simulink model "SupervisorB2"  (R2024b)
settings: Solver=FixedStepDiscrete  StartTime=0.0  StopTime=10.0  FixedStep=0.02  RelTol=1e-3
settings Model: DataDictionary=B2Sup.sldd  PacingRate=0.100000  Creator=miche  LastModifiedBy=Sterm
settings OptimizationCC: DefaultParameterBehavior=Inlined  EnhancedBackFolding=on  PassReuseOutputArgsAs=Individual arguments  ZeroExternalMemoryAtStartup=off  ZeroInternalMemoryAtStartup=off  OptimizeBlockOrder=speed  DifferentSizesBufferReuse=on  OptimizationCustomize=off  EfficientTunableParamExpr=on
settings DebuggingCC: ParameterTunabilityLossMsg=error
settings SFSimCC: MATLABDynamicMemAlloc=off
settings SFSimCC: SimUserIncludeDirs=|
  | C:\Users\Sterm\Desktop\STM32\workspace\Codice_Rover
  | C:\Users\Sterm\Desktop\STM32\workspace\Codice_Rover\Progetto_Board2\Core\Inc
settings RTWCC: Description=Embedded Coder  SystemTargetFile=ert.tlc  GenCodeOnly=on  TemplateMakefile=ert_default_tmf
settings CodeAppCC: ForceParamTrailComments=on  IgnoreCustomStorageClasses=off  OperatorAnnotations=on  SimulinkDataObjDesc=on  SFDataObjDesc=on  InsertBlockDesc=on
settings ERTTargetCC: TargetLangStandard=C99 (ISO)  GenerateSampleERTMain=on  ERTCustomFileTemplate=example_file_process.tlc

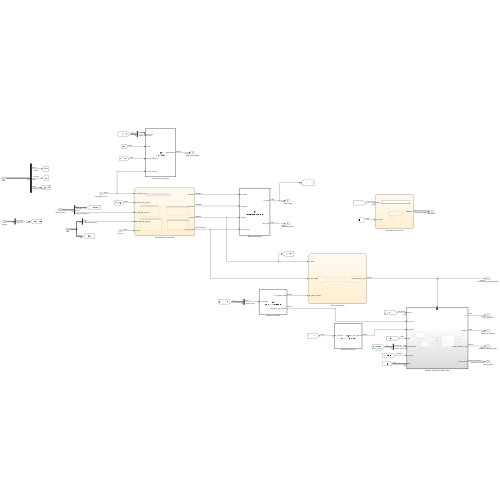
[thumbnail: Simulink's stored preview of the top-level diagram]
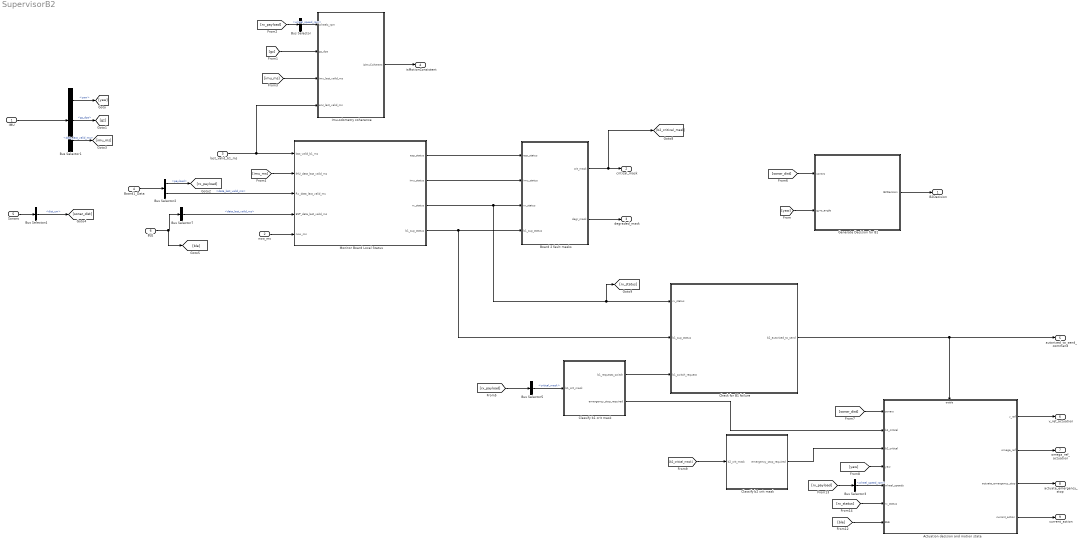
== system SupervisorB2 ==
  IMU : Inport  OutDataTypeStr=Bus: IMUSnapshot_t
  now_ms : Inport  Port=2  OutDataTypeStr=uint32
  last_valid_b1_ms : Inport  Port=3  OutDataTypeStr=uint32
  Board1_Data : Inport  Port=4  OutDataTypeStr=Bus: RxSnapshot_t
  Sonars : Inport  Port=5  OutDataTypeStr=Bus: SonarSnapshot_t
  BLE : Inport  Port=6  OutDataTypeStr=Bus: BleControllerSnapshot_t
  Actuation decision and motion state : Subsystem  TreatAsAtomicUnit=on
  Board 2 fault masks : MATLAB Function  TreatAsAtomicUnit=on
  Bus Selector : BusSelector  OutputSignals=wheel_speed_rpm
  Bus Selector1 : BusSelector  OutputSignals=yaw,gz_dps,data_last_valid_ms
  Bus Selector2 : BusSelector  OutputSignals=payload,data_last_valid_ms
  Bus Selector3 : BusSelector  OutputSignals=wheel_speed_rpm
  Bus Selector4 : BusSelector  OutputSignals=dist_cm
  Bus Selector5 : BusSelector  OutputSignals=critical_mask
  Bus Selector7 : BusSelector  OutputSignals=data_last_valid_ms
  Check for B1 failure : Stateflow chart  TreatAsAtomicUnit=on
      settings: RTWFcnNameOpts=Use subsystem name  RTWFileNameOpts=Use subsystem name  PortSchema="{\"entries\":[{\"content\":{\"sides\":[{\"content\":{\"connectorIds\":[\"In2\",\"In3\",\"In1\"]},\"type\":\"ConnectorPlacement.EquallySpacedRectSide\",\"uuid\":\"67b49e78-6b94-400e-9fcc-b30b67a80691\"},{\"content\":{\"connectorIds\":[\"Out1\"],\"side\":\"RIGHT\"},\"type\":\"ConnectorPlacement.EquallySpacedRectSide\",\"uuid\":\"f9efb856-d575-4b84-9867-a72704ddd64e\"},{\"content\":{\"side\":\"TOP\"},\"type\":\"ConnectorPlacement.EquallySpacedRectSide\",\"uuid\":\"fb0179cd-4de4-48aa-8472-d7b382cb3b22\"}]},\"type\":\"ConnectorPlacement.EquallySpacedConnector\",\"uuid\":\"a3077d23-e6fe-47c9-9a8f-de3eab952316\"}],\"packageUris\":[\"http://schema.mathworks.com/mf0/Connector/R2020b\"],\"version\":\"1.0\"}"
  Classify b1 crit mask : MATLAB Function  TreatAsAtomicUnit=on
  Classify b2 crit mask : MATLAB Function  TreatAsAtomicUnit=on
  Generate Decision for B1 : Stateflow chart  TreatAsAtomicUnit=on
      settings: RTWFcnNameOpts=Use subsystem name  RTWFileNameOpts=Use subsystem name
  Imu-odometry coherence : MATLAB Function  TreatAsAtomicUnit=on
  Monitor Board Local Status : Stateflow chart  TreatAsAtomicUnit=on
      settings: PortSchema="{\"entries\":[{\"content\":{\"sides\":[{\"content\":{\"connectorIds\":[\"In3\",\"In1\",\"In4\",\"In5\",\"In2\"]},\"type\":\"ConnectorPlacement.EquallySpacedRectSide\",\"uuid\":\"47aaac17-a3c1-4cfa-9019-2fc909ce8afb\"},{\"content\":{\"connectorIds\":[\"Out4\",\"Out2\",\"Out3\",\"Out1\"],\"side\":\"RIGHT\"},\"type\":\"ConnectorPlacement.EquallySpacedRectSide\",\"uuid\":\"50480d75-ffb6-4b14-98f4-247cb8499fa0\"},{\"content\":{\"side\":\"TOP\"},\"type\":\"ConnectorPlacement.EquallySpacedRectSide\",\"uuid\":\"1cb4b11b-b488-43f8-b4d2-41a29965dbbd\"}]},\"type\":\"ConnectorPlacement.EquallySpacedConnector\",\"uuid\":\"f85d8103-6e2e-468d-83b6-a974a06ba402\"}],\"packageUris\":[\"http://schema.mathworks.com/mf0/Connector/R2020b\"],\"version\":\"1.0\"}"
  B2Decision : Outport  OutDataTypeStr=Enum: SupervisorCommand_t  PortDimensions=1
  critical_mask : Outport  Port=2  OutDataTypeStr=uint32
  degraded_mask : Outport  Port=3  OutDataTypeStr=uint32
  isMotionConsistent : Outport  Port=4  OutDataTypeStr=boolean
  autorized_to_send_command : Outport  Port=5  OutDataTypeStr=boolean  PortDimensions=1
  v_ref_actuation : Outport  Port=6  OutDataTypeStr=single  PortDimensions=1
  omega_ref_actuation : Outport  Port=7  OutDataTypeStr=single  PortDimensions=1
  actuate_emergency_stop : Outport  Port=8  OutDataTypeStr=boolean
  current_action : Outport  Port=9  OutDataTypeStr=Enum: SupervisorCommand_t
  wires:
  Bus Selector1/1 -> [yaw]  "<yaw>"
  Board1_Data/1 -> Bus Selector2/1
  Bus Selector2/2 -> Monitor Board Local Status/4(Rx_data_last_valid_ms)  "<data_last_valid_ms>"
  Generate Decision for B1/1(B2Decision) -> B2Decision/1
  Monitor Board Local Status/2(imu_status) -> Board 2 fault masks/2(imu_status)
  last_valid_b1_ms/1 -> Monitor Board Local Status/3(last_valid_b1_ms), Imu-odometry coherence/4(enc_last_valid_ms)
  now_ms/1 -> Monitor Board Local Status/2(now_ms)
  Board 2 fault masks/1(crit_mask) -> [b2_critical_mask], critical_mask/1
  IMU/1 -> Bus Selector1/1
  Imu-odometry coherence/1(isImuCoherent) -> isMotionConsistent/1
  [sonar_dist] -> Generate Decision for B1/1(sonars)
  Monitor Board Local Status/1(b1_sup_status) -> Check for B1 failure/3(b1_sup_status), Board 2 fault masks/4(b1_sup_status)
  [yaw] -> Generate Decision for B1/2(gyro_angle)
  Board 2 fault masks/2(degr_mask) -> degraded_mask/1
  Bus Selector1/2 -> [gz]  "<gz_dps>"
  Monitor Board Local Status/4(esp_status) -> Board 2 fault masks/1(esp_status)
  Monitor Board Local Status/3(rx_status) -> Check for B1 failure/2(rx_status), [rx_status], Board 2 fault masks/3(rx_status)
  [gz] -> Imu-odometry coherence/2(gz_dps)
  [rx_payload] -> Bus Selector/1
  Bus Selector1/3 -> [imu_ms]  "<data_last_valid_ms>"
  [imu_ms] -> Imu-odometry coherence/3(imu_last_valid_ms)
  [imu_ms] -> Monitor Board Local Status/1(IMU_data_last_valid_ms)
  Bus Selector2/1 -> [rx_payload]  "<payload>"
  Bus Selector/1 -> Imu-odometry coherence/1(wheels_rpm)  "<wheel_speed_rpm>"
  [rx_payload] -> Bus Selector5/1
  Bus Selector5/1 -> Classify b1 crit mask/1(b1_crit_mask)  "<critical_mask>"
  Classify b1 crit mask/1(b1_requests_switch) -> Check for B1 failure/1(b1_switch_request)
  Classify b1 crit mask/2(emergency_stop_required) -> Actuation decision and motion state/2(b1_critical)
  Check for B1 failure/1(b2_autorized_to_send) -> Actuation decision and motion state/Enable, autorized_to_send_command/1
  Sonars/1 -> Bus Selector4/1
  Bus Selector4/1 -> [sonar_dist]  "<dist_cm>"
  [sonar_dist] -> Actuation decision and motion state/1(sonars)
  [yaw] -> Actuation decision and motion state/4(yaw)
  BLE/1 -> [ble], Bus Selector7/1
  Bus Selector7/1 -> Monitor Board Local Status/5(ESP_data_last_valid_ms)  "<data_last_valid_ms>"
  [ble] -> Actuation decision and motion state/7(BLE)
  [b2_critical_mask] -> Classify b2 crit mask/1(b2_crit_mask)
  Classify b2 crit mask/1(emergency_stop_required) -> Actuation decision and motion state/3(b2_critical)
  Actuation decision and motion state/1(v_ref) -> v_ref_actuation/1
  Actuation decision and motion state/2(omega_ref) -> omega_ref_actuation/1
  Bus Selector3/1 -> Actuation decision and motion state/5(wheel_speeds)  "<wheel_speed_rpm>"
  [rx_payload] -> Bus Selector3/1
  [rx_status] -> Actuation decision and motion state/6(rx_status)
  Actuation decision and motion state/3(actuate_emergency_stop) -> actuate_emergency_stop/1
  Actuation decision and motion state/4(current_action) -> current_action/1

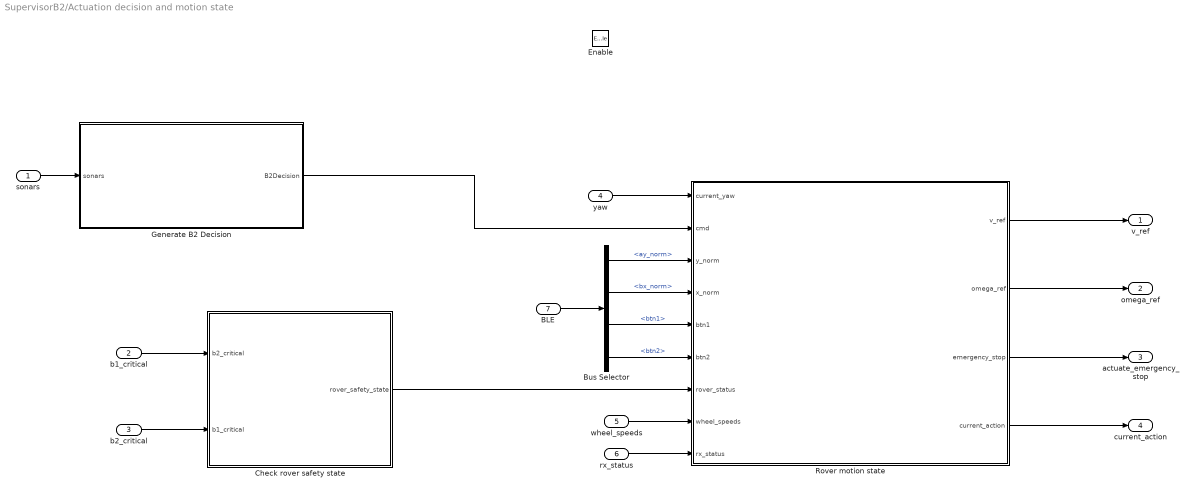
== system SupervisorB2/Actuation decision and motion state ==
  sonars : Inport
  b1_critical : Inport  Port=2
  b2_critical : Inport  Port=3
  yaw : Inport  Port=4
  wheel_speeds : Inport  Port=5
  rx_status : Inport  Port=6
  BLE : Inport  Port=7
  Enable : EnablePort
  Bus Selector : BusSelector  OutputSignals=ay_norm,bx_norm,btn1,btn2
  Check rover safety state : Stateflow chart  TreatAsAtomicUnit=on
      settings: PortSchema="{\"entries\":[{\"content\":{\"sides\":[{\"content\":{\"connectorIds\":[\"In2\",\"In1\"]},\"type\":\"ConnectorPlacement.EquallySpacedRectSide\",\"uuid\":\"9dc33dbe-e010-4406-a301-8909eb6c65d2\"},{\"content\":{\"connectorIds\":[\"Out1\"],\"side\":\"RIGHT\"},\"type\":\"ConnectorPlacement.EquallySpacedRectSide\",\"uuid\":\"084d7bfb-fdfa-425b-9b48-9ea13f8992e6\"},{\"content\":{\"side\":\"TOP\"},\"type\":\"ConnectorPlacement.EquallySpacedRectSide\",\"uuid\":\"e02a7452-bac4-4562-b32b-e5d8b54b8354\"}]},\"type\":\"ConnectorPlacement.EquallySpacedConnector\",\"uuid\":\"22e5b97d-2191-437a-a89c-d8bb13bb1f1c\"}],\"packageUris\":[\"http://schema.mathworks.com/mf0/Connector/R2020b\"],\"version\":\"1.0\"}"
  Generate B2 Decision : Stateflow chart  TreatAsAtomicUnit=on
      settings: RTWFcnNameOpts=Use subsystem name  RTWFileNameOpts=Use subsystem name
  Rover motion state : Stateflow chart  TreatAsAtomicUnit=on
      settings: PortSchema="{\"entries\":[{\"content\":{\"sides\":[{\"content\":{\"connectorIds\":[\"In2\",\"In1\",\"In5\",\"In4\",\"In8\",\"In9\",\"In6\",\"In3\",\"In7\"]},\"type\":\"ConnectorPlacement.EquallySpacedRectSide\",\"uuid\":\"ab2cffc6-18c1-4b62-a79f-6b348f0e6e12\"},{\"content\":{\"connectorIds\":[\"Out2\",\"Out1\",\"Out3\",\"Out4\"],\"side\":\"RIGHT\"},\"type\":\"ConnectorPlacement.EquallySpacedRectSide\",\"uuid\":\"a6f1ea66-886a-456c-a684-893d1155cc5f\"},{\"content\":{\"side\":\"TOP\"},\"type\":\"ConnectorPlacement.EquallySpacedRectSide\",\"uuid\":\"8507e94f-e138-4434-ac51-1bc550838c0e\"}]},\"type\":\"ConnectorPlacement.EquallySpacedConnector\",\"uuid\":\"3184930e-9ebc-43d7-b63a-062e80318630\"}],\"packageUris\":[\"http://schema.mathworks.com/mf0/Connector/R2020b\"],\"version\":\"1.0\"}"
  v_ref : Outport  OutDataTypeStr=single
  omega_ref : Outport  Port=2  OutDataTypeStr=single
  actuate_emergency_stop : Outport  Port=3  OutDataTypeStr=boolean
  current_action : Outport  Port=4  OutDataTypeStr=Enum: SupervisorCommand_t
  wires:
  sonars/1 -> Generate B2 Decision/1(sonars)
  Generate B2 Decision/1(B2Decision) -> Rover motion state/1(cmd)
  Check rover safety state/1(rover_safety_state) -> Rover motion state/6(rover_status)
  Rover motion state/2(v_ref) -> v_ref/1
  Rover motion state/1(omega_ref) -> omega_ref/1
  b1_critical/1 -> Check rover safety state/2(b2_critical)
  b2_critical/1 -> Check rover safety state/1(b1_critical)
  yaw/1 -> Rover motion state/2(current_yaw)
  wheel_speeds/1 -> Rover motion state/3(wheel_speeds)
  rx_status/1 -> Rover motion state/7(rx_status)
  Rover motion state/3(emergency_stop) -> actuate_emergency_stop/1
  Rover motion state/4(current_action) -> current_action/1
  BLE/1 -> Bus Selector/1
  Bus Selector/4 -> Rover motion state/9(btn2)  "<btn2>"
  Bus Selector/3 -> Rover motion state/8(btn1)  "<btn1>"
  Bus Selector/2 -> Rover motion state/4(x_norm)  "<bx_norm>"
  Bus Selector/1 -> Rover motion state/5(y_norm)  "<ay_norm>"

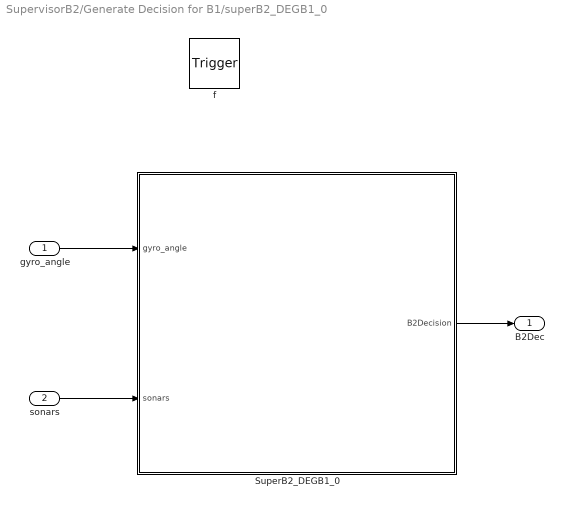
== system SupervisorB2/Generate Decision for B1/superB2_DEGB1_0 ==
  gyro_angle : Inport  OutDataTypeStr=single  PortDimensions=1
  sonars : Inport  Port=2  OutDataTypeStr=uint16  PortDimensions=[1 3]
  f : TriggerPort  TriggerType=function-call  VariantControl=(inherit)
      settings: CopyFcn=Stateflow.SLINSF.SimulinkMan.removeBlockPreDeleteFcn  PreDeleteFcn=Stateflow.SLINSF.SimulinkMan.unsafePredeleteFcn
  SuperB2_DEGB1_0 : Stateflow chart  TreatAsAtomicUnit=on
  B2Dec : Outport  OutDataTypeStr=Enum: SupervisorCommand_t  PortDimensions=1
  wires:
  gyro_angle/1 -> SuperB2_DEGB1_0/1(gyro_angle)
  sonars/1 -> SuperB2_DEGB1_0/2(sonars)
  SuperB2_DEGB1_0/1(B2Decision) -> B2Dec/1

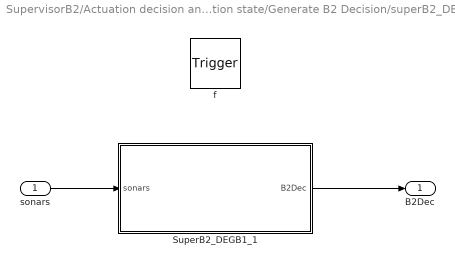
== system SupervisorB2/Actuation decision and motion state/Generate B2 Decision/superB2_DEGB1_1 ==
  sonars : Inport  OutDataTypeStr=uint16  PortDimensions=[1 3]
  f : TriggerPort  TriggerType=function-call  VariantControl=(inherit)
      settings: CopyFcn=Stateflow.SLINSF.SimulinkMan.removeBlockPreDeleteFcn  PreDeleteFcn=Stateflow.SLINSF.SimulinkMan.unsafePredeleteFcn
  SuperB2_DEGB1_1 : Stateflow chart  TreatAsAtomicUnit=on
  B2Dec : Outport  OutDataTypeStr=Enum: SupervisorCommand_t  PortDimensions=1
  wires:
  sonars/1 -> SuperB2_DEGB1_1/1(sonars)
  SuperB2_DEGB1_1/1(B2Dec) -> B2Dec/1

== stateflow chart SupervisorB2/Actuation decision and motion state/Rover motion state ==
  state Backward_mode_toggle [parallel]
    settings: executionOrder=1
    state Combo_toggle_backward
      state Step2
      state Step3
      state Step4
      Step2 -> Step3 [order 1] : [ rising(btn1)]
      Step2 -> (junction 943) [order 2] : [after(1,sec)]
      Step3 -> (junction 943) [order 2] : [after(1,sec)]
      Step3 -> Step4 [order 1] : [rising(btn2)]
      Step4 -> (junction 943) [order 2] : [after(1,sec)]
    state Combo_starting_point
    Combo_starting_point -> Step2 : [rising(btn1) && x_norm == 0 && y_norm == 0]
    (default) -> Combo_starting_point : {backward_enabled = false;}
    Combo_toggle_backward -> Combo_starting_point : [x_norm ~= 0 || y_norm ~= 0]
    (junction 943) -> Combo_starting_point
    (junction 933) -> Combo_starting_point
    Step4 -> (junction 934) [order 1] : [rising(btn2)]
    (junction 934) -> (junction 933) : {backward_enabled = ~backward_enabled}
  state Motion_Supervision [parallel]
    settings: executionOrder=2
    state Stato_marcia_rover
      en,du:
      [V_MAX, OMEGA_MAX] = updateSafetyLimits(rover_status);
      v_user     = y_norm * V_MAX;
      omega_user = x_norm * OMEGA_MAX;
      if invert_y
      if v_user >= 0
      invert_y = false;
      else
      v_user = -v_user;
      end
      end
      ex:
      invert_y = false;
      state Normale_marcia
        en:
        current_action = CMD_NORMAL;
        du:
        if backward_enabled || y_norm > 0
        v_ref = v_user;
        omega_ref = omega_user;
        else
        v_ref = 0;
        omega_ref = omega_user;
        end
      state Retromarcia_180
        en:
        current_action = CMD_ROTATE_180;
        is_rotating180 = true;
        targetAngle = angleCalculator180(current_yaw);
        angle_err = angleError(current_yaw, targetAngle)
        du:
        angle_err = angleError(current_yaw, targetAngle)
        if abs(angle_err) > 45
        omega_ref = sign(-angle_err) *OMEGA_MAX;
        end
        ex:
        is_rotating180 = false;
      (junction 981) -> (junction 991) [order 1] : [v_user < 0]
          | {invert_y = true;}
      (junction 991) -> (junction 974)
      (junction 981) -> (junction 974) [order 2]
      (junction 974) -> Normale_marcia
      Retromarcia_180 -> (junction 981) : [abs(angle_err) < 7.5]
      Normale_marcia -> Retromarcia_180 : [y_norm < -0.5 && ~backward_enabled]
      (default) -> Normale_marcia
    state Procedura_emergency_stop
      state Motori_fermi
        en:
        current_action = CMD_STOP;
        estop_recover_enabled = true;
      state In_frenata_di_emergenza
        en:
        current_action = CMD_ESTOP;
        v_ref = 0;
        omega_ref = 0;
        emergency_stop = true;
        du:
        roverIsStopped = checkStop(wheel_speeds)
      (junction 966) -> Motori_fermi
      (junction 967) -> (junction 966) [order 2] : [duration(roverIsStopped) > 1]
      In_frenata_di_emergenza -> (junction 967)
      (junction 967) -> (junction 964) [order 1] : [rx_status == RX_CRITICAL]
      (junction 964) -> Motori_fermi : [after(2,sec)]
    Stato_marcia_rover -> In_frenata_di_emergenza : [(cmd == CMD_ESTOP && v_user > 0 && ~is_rotating180) || rover_status == SAFETY_CRITICAL]
        | {
        | estop_recover_enabled = false;
        | }
    (default) -> Stato_marcia_rover
    Procedura_emergency_stop -> Stato_marcia_rover : [rover_status ~= SAFETY_CRITICAL && estop_recover_enabled]
        | {
        | emergency_stop = false;
        | }
  data: gyro_angle function_input; targetAngle function_output; gyro_angle function_input; targetAngle function_input; angle_err function_output; rover_state function_input; V_MAX function_output; OMEGA_MAX function_output; wheel_speeds function_input; stop function_output; cmd input Enum: SupervisorCommand_t; current_yaw input; wheel_speeds input; omega_ref output; angle_err local; roverIsStopped local =false; targetAngle local; x_norm input; y_norm input; OMEGA_MAX local; V_MAX local; is_rotating180 local; v_user local; omega_user local; v_ref output; rover_status input Enum: SafetyStatus; invert_y local; emergency_stop output; current_action output Enum: SupervisorCommand_t; rx_status input Enum: RxStatus; estop_recover_enabled local; btn1 input; btn2 input; backward_enabled local
  function targetAngle = angleCalculator180(gyro_angle):
    | function targetAngle = angleCalculator180(gyro_angle)
    | 
    |     angle = gyro_angle + 180;
    |     if angle > 360
    |         targetAngle = angle - 360;
    |     else
    |         targetAngle = angle;
    |     end
    | end
  function angle_err = angleError(gyro_angle, targetAngle):
    | function angle_err = angleError(gyro_angle, targetAngle)
    |     % errore in gradi, range [-180, +180]
    |     angle_err = mod(targetAngle - gyro_angle + 180, 360) - 180;
    | end
  function [V_MAX, OMEGA_MAX] = updateSafetyLimits(rover_state):
    | function [V_MAX, OMEGA_MAX] = updateSafetyLimits(rover_state)
    | 
    | % ---- valori nominali (velocità dimezzata perchè board 2 attua solo se b1
    | % fallisce: quindi di default lo stato è degradato) ----
    | V_MAX          = 0.5;
    | OMEGA_MAX      = 0.5;
    | 
    | if rover_state == SafetyStatus.SAFETY_CRITICAL
    |     V_MAX          = 0;
    |     OMEGA_MAX      = 0;
    | end
    | 
    | end
  function stop = checkStop(wheel_speeds):
    | function stop = checkStop(wheel_speeds)
    | 
    | 
    | stop = all(abs(wheel_speeds(1:4)) < 2.5);
    | 
    | end

== stateflow chart SupervisorB2/Generate Decision for B1 ==
  state B2Dec = superB2_DEGB1_0(gyro_angle,sonars) [function]
  state SuperB2GenerateDecision
  (default) -> SuperB2GenerateDecision
  SuperB2GenerateDecision -> SuperB2GenerateDecision : {B2Decision = superB2_DEGB1_0(gyro_angle, sonars) }
  data: B2Dec function_output Enum: SupervisorCommand_t size=1; gyro_angle function_input single size=1; sonars function_input uint16 size=[1 3]; sonars input size=[1 3]; B2Decision output Enum: SupervisorCommand_t size=1; gyro_angle input single size=1

== stateflow chart SupervisorB2/Check for B1 failure ==
  state B1_actuating
    en:
    b2_autorized_to_send = false;
  state B2_trying_to_actuate
    en:
    b2_autorized_to_send = true;
  B1_actuating -> B2_trying_to_actuate : [b1_switch_request || (rx_status == RX_CRITICAL) || (b1_sup_status == SUPERVISOR_CRITICAL)]
  (default) -> B1_actuating
  B2_trying_to_actuate -> B1_actuating : [duration(~b1_switch_request && rx_status ~= RX_CRITICAL && b1_sup_status ~= SUPERVISOR_CRITICAL) > 3]
  data: b1_switch_request input; rx_status input Enum: RxStatus; b1_sup_status input Enum: SupervisorStatus; b2_autorized_to_send output

== stateflow chart SupervisorB2/Actuation decision and motion state/Generate B2 Decision ==
  state B2Dec = superB2_DEGB1_1(sonars) [function]
  state SuperB2GenerateDecision
  (default) -> SuperB2GenerateDecision
  SuperB2GenerateDecision -> SuperB2GenerateDecision : {B2Decision = superB2_DEGB1_1(sonars) }
  data: sonars function_input uint16 size=[1 3]; B2Dec function_output Enum: SupervisorCommand_t size=1; sonars input size=[1 3]; B2Decision output Enum: SupervisorCommand_t size=1

== stateflow chart SupervisorB2/Actuation decision and motion state/Check rover safety state ==
  state Rover_Degraded_State
    en:
    rover_safety_state = SAFETY_DEGRADED;
  state Rover_Critical_State
    en:
    rover_safety_state = SAFETY_CRITICAL;
  Rover_Critical_State -> Rover_Degraded_State : [~b2_critical && ~b1_critical]
  (default) -> Rover_Degraded_State
  Rover_Degraded_State -> Rover_Critical_State : [b1_critical || b2_critical]
  data: rover_safety_state output Enum: SafetyStatus; b1_critical input; b2_critical input

== matlab function SupervisorB2/Imu-odometry coherence ==
  data: isImuCoherent output; wheels_rpm input; gz_dps input; imu_last_valid_ms input; enc_last_valid_ms input
function isImuCoherent = yawConsistency( ...
        wheels_rpm, gz_dps, imu_last_valid_ms, enc_last_valid_ms)
%#codegen


% PARAMETRI FISICI
r = 0.07;      % [m]
L = 0.38;      % [m]
yaw_correction_factor = 0.83;        %fattore di correzione causa attrito (odometria mostra più rotazione di quella reale)


% PARAMETRI DIAGNOSTICA
WIN_MS  = 100;                 % finestra [ms]
HIST_MS = 1000;                % memoria [ms]
NWIN    = int32(HIST_MS / WIN_MS);

IMU_ENABLE_DTH = deg2rad(1.0); % IMU deve muoversi almeno 1 grado per attivre la diagnostica
ERR_DTH        = deg2rad(1.0); % errore minimo significativo tra IMU e ODOM (per finestra)

HIT_TO_FAULT   = int32(8);     % 8 finestre su 10 -> fault


LONG_WIN_MS = 3000;          %Durata finestra lunga (per errori lenti come deriva)
LONG_ERR_DTH = deg2rad(5);   % 5° errore accumulato


% STATO PERSISTENTE
persistent last_enc_ms last_imu_ms ...
           acc_enc acc_imu ...
           win_start_ms init ...
           hist_hit hist_idx ...
           acc_enc_long acc_imu_long long_start_ms

if isempty(init)
    last_enc_ms    = enc_last_valid_ms;
    last_imu_ms    = imu_last_valid_ms;
    acc_enc        = 0.0;
    acc_imu        = 0.0;
    win_start_ms   = imu_last_valid_ms;

    hist_hit       = zeros(1, double(NWIN), 'int32');
    hist_idx       = int32(1);

    acc_enc_long = 0.0;
    acc_imu_long = 0.0;
    long_start_ms = imu_last_valid_ms;

    init = true;
end

isImuCoherent = true;


% ODOMETRIA
rpm_L = 0.5 * (wheels_rpm(1) + wheels_rpm(3));
rpm_R = 0.5 * (wheels_rpm(2) + wheels_rpm(4));

K = 2*pi*r / (60*L);
omega_enc = yaw_correction_factor * K * double(rpm_L - rpm_R);   % [rad/s]


% CALCOLO YAW CON ODOMETRIA (integrando accellerazione stimata)
if enc_last_valid_ms ~= last_enc_ms
    dt = double(enc_last_valid_ms - last_enc_ms) * 1e-3;
    last_enc_ms = enc_last_valid_ms;
    if dt > 0 && dt < 0.1
        acc_enc = acc_enc + omega_enc * dt;
        acc_enc_long = acc_enc_long + omega_enc * dt;
    end
end


% INTEGRA YAW CON IMU (integrando gz)
if imu_last_valid_ms ~= last_imu_ms
    dt = double(imu_last_valid_ms - last_imu_ms) * 1e-3;
    last_imu_ms = imu_last_valid_ms;
    if dt > 0 && dt < 0.1
        omega_imu = double(gz_dps) * pi/180;   % [rad/s]
        acc_imu = acc_imu + omega_imu * dt;
        acc_imu_long = acc_imu_long + omega_imu * dt;
    end
end



% FINE FINESTRA VELOCE
if (imu_last_valid_ms - win_start_ms) >= WIN_MS

    hist_hit(hist_idx) = int32(0);
    % diagnostica disattivata se IMU praticamente ferma
    if abs(acc_imu) >= IMU_ENABLE_DTH

        err = acc_imu - acc_enc;

        if abs(err) >= ERR_DTH
            hist_hit(hist_idx) = int32(1);
        end
    end

    % decisione su ultimo ~1s
    total_window_hits = int32(sum(hist_hit));

    %Se più di HIT_TO_FAULT (8 in questo caso) finestre presentano errore
    %allora diciamo che c'è discrepanza tra imu e odometria (possibile fault motore) 
    if total_window_hits >= HIT_TO_FAULT
        isImuCoherent = false;
    else
        isImuCoherent = true;
    end

    % reset finestra
    acc_enc      = 0.0;
    acc_imu      = 0.0;
    win_start_ms = imu_last_valid_ms;

    hist_idx = hist_idx + 1;
    if hist_idx > NWIN
        hist_idx = int32(1);
    end
end

% FINESTRA LUNGA (usata per errori lenti come deriva quando si prova ad
% andare avanti senza sterzare)
if (imu_last_valid_ms - long_start_ms) >= LONG_WIN_MS
    
    long_err = acc_imu_long - acc_enc_long;

    if abs(long_err) >= LONG_ERR_DTH
        isImuCoherent = false;
    end

    acc_enc_long = 0.0;
    acc_imu_long = 0.0;
    long_start_ms = imu_last_valid_ms;

end

end

== matlab function SupervisorB2/Classify b1 crit mask ==
  data: b1_crit_mask input; b1_requests_switch output; emergency_stop_required output
function [ ...
    b1_requests_switch, ...   % bool
    emergency_stop_required ...% bool
] = classifyB1CriticalMask(b1_crit_mask)
%#codegen

b1_crit_mask = uint32(b1_crit_mask);

% --- bit definitions ---
RX_BIT    = uint32(2);
B2SUP_BIT = uint32(7);

RX_MASK    = bitshift(uint32(1), RX_BIT);
B2SUP_MASK = bitshift(uint32(1), B2SUP_BIT);

SWITCH_MASK = bitor(RX_MASK, B2SUP_MASK);

% --- critical che abilitano switch board ---
b1_switch_mask = bitand(b1_crit_mask, SWITCH_MASK);
b1_requests_switch = (b1_switch_mask ~= 0);

% --- altri critical (quelli che fermano il rover) ---
b1_other_crit_mask = bitand( ...
    b1_crit_mask, ...
    bitcmp(SWITCH_MASK, 'uint32') ...
);

emergency_stop_required = (b1_other_crit_mask ~= 0);

== stateflow chart SupervisorB2/Actuation decision and motion state/Generate B2 Decision/superB2_DEGB1_1/SuperB2_DEGB1_1 ==
  state check_sonars_for_moving_again
    en:
    % fermati
    B2Dec = CMD_ESTOP;
  state check_sonars_for_stopping
    en:
    % muoviti in modalità degradata
    B2Dec  = CMD_NORMAL;
  (default) -> check_sonars_for_stopping
  check_sonars_for_stopping -> check_sonars_for_moving_again : [check_emergency_stop(sonars)]
  check_sonars_for_moving_again -> check_sonars_for_stopping : [~check_emergency_stop(sonars)]
  data: sonars function_input; stop function_output uint8 size=1; sonars input size=[1 3]; B2Dec output Enum: SupervisorCommand_t size=1
  function stop = check_emergency_stop(sonars):
    | function stop = check_emergency_stop(sonars)
    | 
    | s1 = sonars(1);
    | s2 = sonars(2);
    | s3 = sonars(3);
    | 
    | % se aLmeno un sonar rileva un ostacolo ad una distanza inferiore a 70cm, 
    | % fermati 
    | if(s1<300 || s2<300 || s3<00)
    |     stop = uint8(1);
    | else
    |     stop = uint8(0);
    | end
    | 
    | end

== matlab function SupervisorB2/Classify b2 crit mask ==
  data: b2_crit_mask input; emergency_stop_required output
function emergency_stop_required = classifyB2CriticalMask(b2_crit_mask)
%#codegen


% --- bit definitions ---
ESP_BIT    = uint32(0);
IMU_BIT = uint32(1);

ESP_MASK    = bitshift(uint32(1), ESP_BIT);
IMU_MASK = bitshift(uint32(1), IMU_BIT);

EMERGENCY_MASK = bitor(ESP_MASK, IMU_MASK);

% --- critical che abilitano switch board ---
b2_emergency_mask = bitand(b2_crit_mask, EMERGENCY_MASK);
emergency_stop_required = (b2_emergency_mask ~= 0);

end

== stateflow chart SupervisorB2/Monitor Board Local Status ==
  state MonitorBLE [parallel]
    settings: executionOrder=2
    state ESP_critical
      en:
      esp_status = ESP_I2C_CRITICAL;
      du:
      degraded_esp = isCommDegradedByMeanPeriod(...
      ESP_data_last_valid_ms, 40);
    state ESP_ok
      en:
      esp_status = ESP_I2C_OK;
      du:
      degraded_esp = isCommDegradedByMeanPeriod(...
      ESP_data_last_valid_ms, 40);
    state ESP_degraded
      en:
      esp_status = ESP_I2C_DEGRADED;
      du:
      degraded_esp = isCommDegradedByMeanPeriod(...
      ESP_data_last_valid_ms, 40);
    ESP_critical -> (junction 712) : [duration(~degraded_esp) > 1]
    (junction 712) -> ESP_ok
    (junction 730) -> ESP_critical
    (junction 715) -> ESP_critical
    ESP_ok -> (junction 730) [order 2] : [now_ms - ESP_data_last_valid_ms > 120]
    ESP_degraded -> (junction 715) [order 2] : [now_ms - ESP_data_last_valid_ms > 120]
    ESP_degraded -> ESP_ok [order 1] : [duration(~degraded_esp) > 1]
    (default) -> ESP_ok
    ESP_ok -> ESP_degraded [order 1] : [degraded_esp]
  state MonitorBoard1Supervisor [parallel]
    settings: executionOrder=1
    state B1_sup_critical
      en:
      b1_sup_status = SUPERVISOR_CRITICAL;
      du:
      degraded_sup = isCommDegradedByMeanPeriod(...
      last_valid_b1_ms, 60);
    state B1_sup_ok
      en:
      b1_sup_status = SUPERVISOR_OK;
      du:
      degraded_sup = isCommDegradedByMeanPeriod(...
      last_valid_b1_ms, 60);
    state B1_sup_degraded
      en:
      b1_sup_status = SUPERVISOR_DEGRADED;
      du:
      degraded_sup = isCommDegradedByMeanPeriod(...
      last_valid_b1_ms, 60);
    B1_sup_critical -> (junction 766) : [duration(~degraded_sup) > 2]
    (junction 766) -> B1_sup_ok
    (junction 765) -> B1_sup_critical
    (junction 764) -> B1_sup_critical
    B1_sup_ok -> (junction 765) [order 2] : [now_ms - last_valid_b1_ms > 150]
    B1_sup_degraded -> (junction 764) [order 2] : [now_ms - last_valid_b1_ms > 150]
    B1_sup_degraded -> B1_sup_ok [order 1] : [duration(~degraded_sup) > 1]
    (default) -> B1_sup_ok
    B1_sup_ok -> B1_sup_degraded [order 1] : [degraded_sup]
  state MonitorIMU [parallel]
    settings: executionOrder=3
    state IMU_critical
      en:
      imu_status = IMU_I2C_CRITICAL;
      du:
      degraded_imu = isCommDegradedByMeanPeriod(...
      IMU_data_last_valid_ms, 100);
    state IMU_ok
      en:
      imu_status = IMU_I2C_OK;
      du:
      degraded_imu = isCommDegradedByMeanPeriod(...
      IMU_data_last_valid_ms, 100);
    state IMU_degraded
      en:
      imu_status = IMU_I2C_DEGRADED;
      du:
      degraded_imu = isCommDegradedByMeanPeriod(...
      IMU_data_last_valid_ms, 100);
    IMU_critical -> (junction 741) : [duration(~degraded_imu) > 1]
    (junction 741) -> IMU_ok
    (junction 742) -> IMU_critical
    (junction 740) -> IMU_critical
    IMU_ok -> (junction 742) [order 2] : [now_ms - IMU_data_last_valid_ms > 200]
    IMU_degraded -> (junction 740) [order 2] : [now_ms - IMU_data_last_valid_ms > 200]
    IMU_degraded -> IMU_ok [order 1] : [duration(~degraded_imu) > 1]
    (default) -> IMU_ok
    IMU_ok -> IMU_degraded [order 1] : [degraded_imu]
  state MonitorRx [parallel]
    settings: executionOrder=4
    state Rx_critical
      en:
      rx_status = RX_CRITICAL;
      du:
      degraded_rx = isCommDegradedByMeanPeriod(...
      Rx_data_last_valid_ms, 40);
    state Rx_ok
      en:
      rx_status = RX_OK;
      du:
      degraded_rx = isCommDegradedByMeanPeriod(...
      Rx_data_last_valid_ms, 40);
    state Rx_degraded
      en:
      rx_status = RX_DEGRADED;
      du:
      degraded_rx = isCommDegradedByMeanPeriod(...
      Rx_data_last_valid_ms, 40);
    Rx_critical -> (junction 780) : [duration(~degraded_rx) > 1]
    (junction 780) -> Rx_ok
    (junction 781) -> Rx_critical
    (junction 782) -> Rx_critical
    Rx_ok -> (junction 781) [order 2] : [now_ms - Rx_data_last_valid_ms > 120]
    Rx_degraded -> (junction 782) [order 2] : [now_ms - Rx_data_last_valid_ms > 120]
    Rx_degraded -> Rx_ok [order 1] : [duration(~degraded_rx) > 1]
    (default) -> Rx_ok
    Rx_ok -> Rx_degraded [order 1] : [degraded_rx]
  data: data_last_valid_ms function_input; mean_threshold_ms function_input; comm_degraded function_output; IMU_data_last_valid_ms input uint32; now_ms input; last_valid_b1_ms input; b1_sup_status output Enum: SupervisorStatus; imu_status output Enum: ImuStatus; Rx_data_last_valid_ms input; rx_status output Enum: RxStatus; degraded_sup local =false; degraded_rx local =false; degraded_imu local =false; degraded_esp local =false; ESP_data_last_valid_ms input; esp_status output Enum: EspStatus
  function comm_degraded = isCommDegradedByMeanPeriod(data_last_valid_ms, mean_threshold_ms):
    | function comm_degraded = isCommDegradedByMeanPeriod(data_last_valid_ms, mean_threshold_ms)
    | % ISCOMMDEGRADEDBYMEANPERIOD
    | % Valuta stato "degraded" in base alla media dei tempi di arrivo dati.
    | %
    | % INPUT:
    | %   data_last_valid_ms   - timestamp ultimo dato valido (ms)
    | %   mean_threshold_ms    - soglia media periodo (ms), es. 100
    | %
    | % OUTPUT:
    | %   comm_degraded        - true se mean_dt > mean_threshold_ms
    | %   mean_dt              - periodo medio stimato (ms)
    | 
    | % ----------------------------
    | % PARAMETRI DI PROGETTO
    | % ----------------------------
    | N_SAMPLES = 10;   % numero di periodi mediati
    | 
    | % ----------------------------
    | % STATO PERSISTENTE
    | % ----------------------------
    | persistent last_valid_prev buf idx count sum_dt
    | 
    | if isempty(last_valid_prev)
    |     last_valid_prev = data_last_valid_ms;
    |     buf   = zeros(1, N_SAMPLES);
    |     idx   = 1;
    |     count = 0;
    |     sum_dt = uint32(0);
    | 
    |     comm_degraded = false;
    |     return;
    | end
    | 
    | % ----------------------------
    | % NUOVO DATO ARRIVATO?
    | % ----------------------------
    | if data_last_valid_ms ~= last_valid_prev
    | 
    |     dt = data_last_valid_ms - last_valid_prev;
    |     last_valid_prev = data_last_valid_ms;
    | 
    |     % Sliding window O(1)
    |     old = buf(idx);
    |     buf(idx) = dt;
    |     sum_dt = sum_dt - old + dt;
    | 
    |     idx = idx + 1;
    |     if idx > N_SAMPLES
    |         idx = 1;
    |     end
    | 
    |     if count < N_SAMPLES
    |         count = count + 1;
    |     end
    | end
    | 
    | % ----------------------------
    | % MEDIA E DECISIONE
    | % ----------------------------
    | if count > 0
    |     mean_dt = sum_dt / count;
    | else
    |     mean_dt = uint32(0);
    | end
    | 
    | comm_degraded = (mean_dt > mean_threshold_ms);
    | 
    | end

== matlab function SupervisorB2/Board 2 fault masks ==
  data: esp_status input Enum: EspStatus; crit_mask output; imu_status input; rx_status input; b1_sup_status input; degr_mask output
function [crit_mask, degr_mask] = buildBoard2FaultMasks( ...
    esp_status, imu_status, rx_status, b1_sup_status)

crit_mask = uint32(0);
degr_mask = uint32(0);

% ---- BLE Controller ----
if esp_status == EspStatus.ESP_I2C_CRITICAL
    crit_mask = bitor(crit_mask, bitshift(uint32(1), 0));
elseif esp_status == EspStatus.ESP_I2C_DEGRADED
    degr_mask = bitor(degr_mask, bitshift(uint32(1), 0));
end

% ---- IMU ----
if imu_status == ImuStatus.IMU_I2C_CRITICAL
    crit_mask = bitor(crit_mask, bitshift(uint32(1), 1));
elseif imu_status == ImuStatus.IMU_I2C_DEGRADED
    degr_mask = bitor(degr_mask, bitshift(uint32(1), 1));
end

% ---- RX ----
if rx_status == RxStatus.RX_CRITICAL
    crit_mask = bitor(crit_mask, bitshift(uint32(1), 2));
elseif rx_status == RxStatus.RX_DEGRADED
    degr_mask = bitor(degr_mask, bitshift(uint32(1), 2));
end

% ---- B1 Supervisor ----
if b1_sup_status == SupervisorStatus.SUPERVISOR_CRITICAL
    crit_mask = bitor(crit_mask, bitshift(uint32(1), 3));
elseif b1_sup_status == SupervisorStatus.SUPERVISOR_DEGRADED
    degr_mask = bitor(degr_mask, bitshift(uint32(1), 3));
end

== stateflow chart SupervisorB2/Generate Decision for B1/superB2_DEGB1_0/SuperB2_DEGB1_0 ==
  note: B2 Decision
      |
      | --- IF DEG_B1 == 0:
      | 0: pronto ad eseguire il comando utente
      | 1: almeno un sonar < 70cm. Stop
      | 2: muoversi in direzione sonar1
      | 3: muoversi in direzione sonar2
      | 4: muoversi in direzione sonar3
  state B2Decisions [parallel]
    settings: executionOrder=1
    state MoveToS3
      en:
      B2Decision = CMD_GO_RIGHT;
      targetAngle= angleCalculator(gyro_angle, B2Decision)
    state Waiting
      en:
      B2Decision = ...
      CMD_NORMAL;
    state AvoidS1
      en:
      B2Decision = ...
      CMD_AVOID_LEFT;
    state AvoidS3
      en:
      B2Decision = ...
      CMD_AVOID_RIGHT;
    state MoveToS1
      en:
      B2Decision = CMD_GO_LEFT;
      targetAngle= angleCalculator(gyro_angle, B2Decision)
    state InEmergency
      entry:
      B2Decision = ...
      CMD_ESTOP;
    MoveToS3 -> (junction 54) [order 1] : emergency
    B2Decisions.Waiting -> (junction 54) [order 1] : emergency
    AvoidS3 -> (junction 54) [order 1] : emergency
    (junction 54) -> InEmergency
    MoveToS3 -> B2Decisions.Waiting [order 2] : [gyroTargetDiff(gyro_angle, targetAngle)]
    B2Decisions.Waiting -> MoveToS3 [order 2] : moveToS3
    (default) -> B2Decisions.Waiting
    AvoidS3 -> B2Decisions.Waiting [order 2] : [after(0.5,  sec)]
    AvoidS1 -> B2Decisions.Waiting [order 2] : [after(0.5,  sec)]
    B2Decisions.Waiting -> AvoidS3 [order 3] : avoidS3
    B2Decisions.Waiting -> AvoidS1 [order 5] : avoidS1
    InEmergency -> B2Decisions.Waiting : safe
    AvoidS1 -> (junction 42) [order 1] : emergency
    MoveToS1 -> B2Decisions.Waiting [order 2] : [gyroTargetDiff(gyro_angle, targetAngle)]
    B2Decisions.Waiting -> MoveToS1 [order 4] : moveToS1
    (junction 7) -> InEmergency
    MoveToS1 -> (junction 48) [order 1] : emergency
    (junction 42) -> (junction 48)
    (junction 48) -> (junction 7)
  state Sonars [parallel]
    settings: executionOrder=2
    state distance_70 [parallel]
      settings: executionOrder=1
      state check_sonars_for_moving_again
        en:
        stop = check_emergency_stop(sonars)
        during:
        stop = check_emergency_stop(sonars)
      state check_sonars_for_stopping
        en:
        stop = check_emergency_stop(sonars)
        during:
        stop = check_emergency_stop(sonars)
      (default) -> check_sonars_for_stopping
      check_sonars_for_stopping -> check_sonars_for_moving_again : [stop]{send(emergency, B2Decisions)}
      check_sonars_for_moving_again -> check_sonars_for_stopping : [~stop]{send(safe, B2Decisions)}
    state distance_gt70 [parallel]
      settings: executionOrder=2
      state Waiting_S1 [parallel]
        settings: executionOrder=1
        state WS1
          en:
          isClose1 =closeRange(sonars(1))
          du:
          isClose1 =closeRange(sonars(1))
        (default) -> WS1
        (junction 26) -> WS1
        (junction 15) -> WS1
        (junction 86) -> (junction 26) : {obj1Detected = 0
            | send(Fall1, timers)}
        (junction 33) -> (junction 15) : {obj1Detected = 1 }
        WS1 -> (junction 36) : [~stop]
        (junction 36) -> (junction 33) [order 1] : [isClose1]
        (junction 36) -> (junction 86) [order 2] : [~isClose1 & obj1Detected == 1]
      state Waiting_S2 [parallel]
        settings: executionOrder=2
        state WS2
          en:
          isClose2 =closeRange(sonars(2))
          du:
          isClose2 =closeRange(sonars(2))
        (default) -> WS2
        (junction 65) -> WS2
        (junction 96) -> WS2
        (junction 66) -> (junction 96) : {obj2Detected = 0
            | send(Fall2, timers)}
        (junction 77) -> (junction 65) : {obj2Detected = 1 }
        WS2 -> (junction 58) : [~stop]
        (junction 58) -> (junction 77) [order 1] : [isClose2]
        (junction 58) -> (junction 66) [order 2] : [~isClose2 & obj2Detected == 1]
      state Waiting_S3 [parallel]
        settings: executionOrder=3
        state WS3
          en:
          isClose3 =closeRange(sonars(3))
          du:
          isClose3 =closeRange(sonars(3))
        (default) -> WS3
        (junction 92) -> WS3
        (junction 94) -> WS3
        (junction 95) -> (junction 94) : {obj3Detected = 0
            | send(Fall3, timers)}
        (junction 60) -> (junction 92) : {obj3Detected = 1 }
        WS3 -> (junction 82) : [~stop]
        (junction 82) -> (junction 60) [order 1] : [isClose3]
        (junction 82) -> (junction 95) [order 2] : [~isClose3 & obj3Detected == 1]
    state timers [parallel]
      settings: executionOrder=3
      state timerSonar12 [parallel]
        settings: executionOrder=1
        state Waiting
        state Fall1Detected
        (junction 103) -> (junction 79) : {send(moveToS1, B2Decisions)}
        (junction 79) -> Sonars.timers.timerSonar12.Waiting
        (junction 61) -> (junction 103)
        (default) -> Sonars.timers.timerSonar12.Waiting
        Sonars.timers.timerSonar12.Waiting -> Sonars.timers.timerSonar12.Fall1Detected : Fall1
        Sonars.timers.timerSonar12.Fall1Detected -> (junction 61) [order 2] : [obj2Detected]
        Sonars.timers.timerSonar12.Fall1Detected -> Sonars.timers.timerSonar12.Waiting [order 1] : after(3,sec)
      state timerSonar21 [parallel]
        settings: executionOrder=2
        state Waiting
        state Fall1Detected
        (junction 142) -> (junction 120) : {send(avoidS1, B2Decisions)}
        (junction 120) -> Sonars.timers.timerSonar21.Waiting
        (junction 137) -> (junction 142)
        (default) -> Sonars.timers.timerSonar21.Waiting
        Sonars.timers.timerSonar21.Waiting -> Sonars.timers.timerSonar21.Fall1Detected : Fall2
        Sonars.timers.timerSonar21.Fall1Detected -> (junction 137) [order 2] : [obj1Detected]
        Sonars.timers.timerSonar21.Fall1Detected -> Sonars.timers.timerSonar21.Waiting [order 1] : after(3,sec)
      state timerSonar23 [parallel]
        settings: executionOrder=3
        state Waiting
        state Fall1Detected
        (junction 113) -> (junction 139) : {send(avoidS3, B2Decisions)}
        (junction 139) -> Sonars.timers.timerSonar23.Waiting
        (junction 144) -> (junction 113)
        (default) -> Sonars.timers.timerSonar23.Waiting
        Sonars.timers.timerSonar23.Waiting -> Sonars.timers.timerSonar23.Fall1Detected : Fall2
        Sonars.timers.timerSonar23.Fall1Detected -> (junction 144) [order 2] : [obj3Detected]
        Sonars.timers.timerSonar23.Fall1Detected -> Sonars.timers.timerSonar23.Waiting [order 1] : after(3,sec)
      state timerSonar32 [parallel]
        settings: executionOrder=4
        state Waiting
        state Fall1Detected
        (junction 117) -> (junction 122) : {send(moveToS3, B2Decisions)}
        (junction 122) -> Sonars.timers.timerSonar32.Waiting
        (junction 115) -> (junction 117)
        (default) -> Sonars.timers.timerSonar32.Waiting
        Sonars.timers.timerSonar32.Waiting -> Sonars.timers.timerSonar32.Fall1Detected : Fall3
        Sonars.timers.timerSonar32.Fall1Detected -> (junction 115) [order 2] : [obj2Detected]
        Sonars.timers.timerSonar32.Fall1Detected -> Sonars.timers.timerSonar32.Waiting [order 1] : after(3,sec)
  data: gyro_angle function_input; targetAngle function_input; moved function_output; sonars function_input; stop function_output uint8 size=1; gyro_angle function_input; B2Decision function_input; targetAngle function_output; sonar function_input; isClose function_output uint8 size=1; gyro_angle input single size=1; sonars input size=[1 3]; B2Decision output Enum: SupervisorCommand_t size=1; isClose1 local uint8 size=1 =0; isClose2 local uint8 size=1 =0; isClose3 local uint8 size=1 =0; obj1Detected local uint8 size=1 =0; obj2Detected local uint8 size=1 =0; obj3Detected local uint8 size=1 =0; stop local uint8 size=1 =0; targetAngle local single size=1 =0
  events: Fall1 local FUNCTION_CALL_EVENT; Fall2 local FUNCTION_CALL_EVENT; Fall3 local FUNCTION_CALL_EVENT; emergency local FUNCTION_CALL_EVENT; moveToS1 local FUNCTION_CALL_EVENT; moveToS3 local FUNCTION_CALL_EVENT; safe local FUNCTION_CALL_EVENT; avoidS1 local FUNCTION_CALL_EVENT; avoidS3 local FUNCTION_CALL_EVENT
  function moved = gyroTargetDiff(gyro_angle, targetAngle):
    | function moved = gyroTargetDiff(gyro_angle, targetAngle)
    | 
    | moved = abs(mod(targetAngle - gyro_angle + 180, 360) - 180) < 12;
    | 
    | end
  function stop = check_emergency_stop(sonars):
    | function stop = check_emergency_stop(sonars)
    | 
    | s1 = sonars(1);
    | s2 = sonars(2);
    | s3 = sonars(3);
    | 
    | % se aLmeno un sonar rileva un ostacolo ad una distanza inferiore a 70cm, 
    | % fermati 
    | if(s1<=70 || s2<=70 || s3<=70)
    |     stop = uint8(1);
    | else
    |     stop = uint8(0);
    | end
    | 
    | end
  function targetAngle = angleCalculator(gyro_angle, B2Decision):
    | function targetAngle = angleCalculator(gyro_angle, B2Decision)
    | 
    | if B2Decision == 2              % gira verso sonar 1, quindi in senso antiorario
    |     
    |     angle = gyro_angle - 45;
    |     if angle < 0
    |         targetAngle = 360 + angle;
    |     else
    |         targetAngle = angle;
    |     end
    | 
    | else                            % gira verso sonar 3, quindi in senso orario
    | 
    |     angle = gyro_angle + 45;
    |     if angle > 360
    |         targetAngle = angle - 360;
    |     else
    |         targetAngle = angle;
    |     end
    | end
    | 
    | 
    | 
    | end
  function isClose = closeRange(sonar):
    | function isClose = closeRange(sonar)
    | 
    | 
    | distMinClose = 100;   %per test 75
    | distMaxClose = 300;   %per test 150
    | 
    | 
    | if(sonar > distMinClose && sonar < distMaxClose)
    |     isClose = uint8(1);
    | else
    |     isClose = uint8(0);
    | end
